simulink model "Problem1_Linearized"  (R2018a)
settings: Solver=VariableStepAuto  StartTime=0.0  StopTime=tStop  MaxStep=T/4  RelTol=1e-3
values from neighbouring files (symbols this model uses):
  A1 = [-2*Ron/L -1/L; 1/C -1/(R*C)]    [EE458_HW1_Solution.m]
  B1 = [2*Vg/L (2*D-1)/L; 0 0]    [EE458_HW1_Solution.m]
  d_afterProblem1 = 0.9    [EE458_HW1_Solution.m]
  d_beforeProblem1 = 0.7    [EE458_HW1_Solution.m]
  tStepDuty = 40e-3    (= 0.04)    [EE458_HW1_Solution.m]
  tStepVg = 20e-3    (= 0.02)    [EE458_HW1_Solution.m]
  U = [D; Vg]    [EE458_HW1_Solution.m]
  vg_after = 75    [EE458_HW1_Solution.m]
  vg_before = 100    [EE458_HW1_Solution.m]
  X1 = [I1; V1]    [EE458_HW1_Solution.m]
undefined symbols (not defined in the file or in its folder): plecs
settings Model: Creator=brianbj  LastModifiedBy=brianbj

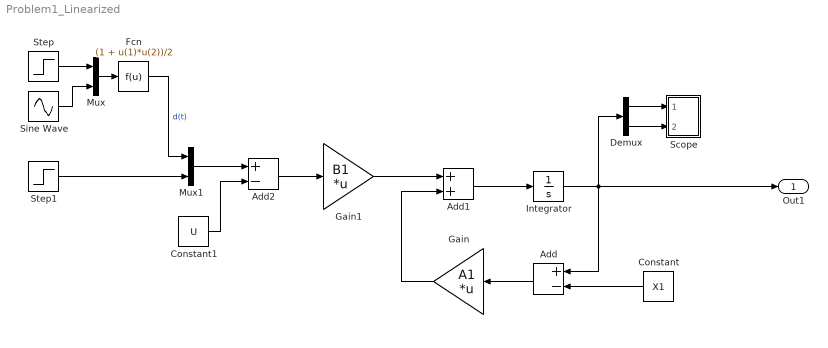
== system Problem1_Linearized ==
  Add : Sum  Inputs=+-
  Add1 : Sum
  Add2 : Sum  Inputs=+-
  Constant : Constant  Value=X1
  Constant1 : Constant  Value=U
  Demux : Demux  Outputs=2
  Fcn : Fcn  Expr=(1 + u(1)*u(2))/2
  Gain : Gain  Gain=A1  Multiplication=Matrix(K*u) (u vector)
  Gain1 : Gain  Gain=B1  Multiplication=Matrix(K*u) (u vector)
  Integrator : Integrator  InitialCondition=X1
  Mux : Mux  Inputs=2
  Mux1 : Mux  Inputs=2
  Scope : Subsystem  LoadFcn=plecs('sl', 300);  InitFcn=plecs('sl', 314);  StartFcn=plecs('sl', 308);  StopFcn=plecs('sl', 309);  mask{Settings=<binary blob, 1188 chars, not shown>}
      mask init:
      | plecs('sl', 315);
      settings: CopyFcn=plecs('sl', 303);  DeleteFcn=plecs('sl', 305);  UndoDeleteFcn=plecs('sl', 306);  PreSaveFcn=plecs('sl', 311);  NameChangeFcn=plecs('sl', 310);  DestroyFcn=plecs('sl', 307);  OpenFcn=plecs('sl', 302);  ErrorFcn=plerrorfcn
      mask Display: plot([0.1 0.9 0.9 0.1 0.1], [0.9 0.9 0.5 0.5 0.9])
  Sine Wave : Sin  Frequency=2*pi*50  SampleTime=0
  Step : Step  Time=tStepDuty  Before=d_beforeProblem1  After=d_afterProblem1  SampleTime=0
  Step1 : Step  Time=tStepVg  Before=vg_before  After=vg_after  SampleTime=0
  Out1 : Outport
  wires:
  Integrator/1 -> Demux/1, Out1/1, Add/1
  Add/1 -> Gain/1
  Add1/1 -> Integrator/1
  Gain1/1 -> Add1/1
  Gain/1 -> Add1/2
  Add2/1 -> Gain1/1
  Constant/1 -> Add/2
  Constant1/1 -> Add2/2
  Step/1 -> Mux/1
  Sine Wave/1 -> Mux/2
  Step1/1 -> Mux1/2
  Mux/1 -> Fcn/1
  Fcn/1 -> Mux1/1  "d(t)"
  Mux1/1 -> Add2/1
  Demux/1 -> Scope/1(1)
  Demux/2 -> Scope/2(2)

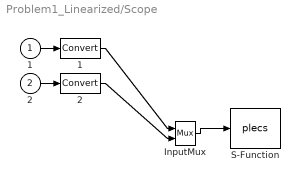
== system Problem1_Linearized/Scope ==
  1 : Inport
  2 : Inport  Port=2
  " 1 " : DataTypeConversion  SaturateOnIntegerOverflow=on  RndMeth=Zero
  " 2 " : DataTypeConversion  SaturateOnIntegerOverflow=on  RndMeth=Zero
  " InputMux " : Mux  Inputs=2
  " S-Function " : S-Function  FunctionName=plecs  SFunctionDeploymentMode=off  EnableBusSupport=off
  wires:
  " InputMux "/1 -> " S-Function "/1
  1/1 -> " 1 "/1
  " 1 "/1 -> " InputMux "/1
  2/1 -> " 2 "/1
  " 2 "/1 -> " InputMux "/2
